simulink model "ProyectoFinal"  (R2024b)
settings: Solver=ode15s  StartTime=0.0  StopTime=10  RelTol=1e-3
undefined symbols (not defined in the file): sigbuilder_block
libraries: slpidlib x1
settings Model: LastModifiedBy=DELL
settings DataIOCC: ReturnWorkspaceOutputs=off  TimeSaveName=t

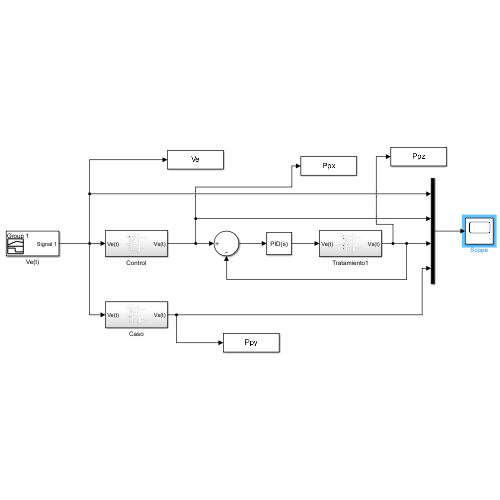
[thumbnail: Simulink's stored preview of the top-level diagram]
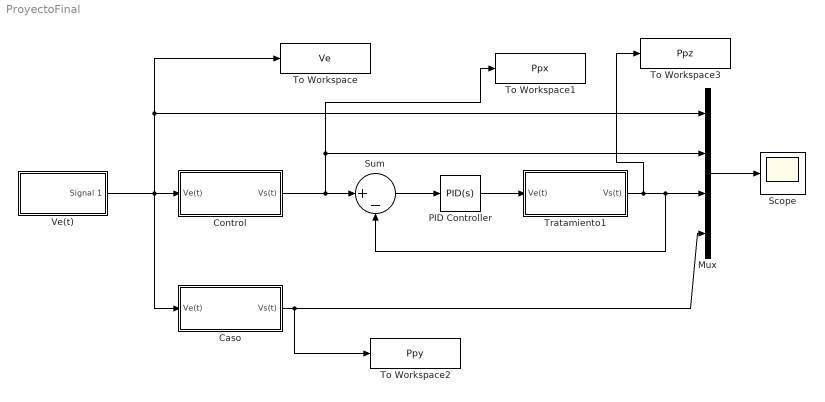
== system ProyectoFinal ==
  Caso : Subsystem
  Control : Subsystem
  Mux : Mux
  PID Controller : slpidlib/PID Controller  Controller=PID  Form=Parallel  TimeDomain=Continuous-time  UseExternalTs=off  SampleTime=-1  IntegratorMethod=Forward Euler  FilterMethod=Forward Euler  ControllerParametersSource=internal  P=8218.94505806436  I=15443765.2569091  UseKiTs=off  D=0.14672186378579  UseExternalDerivativeSource=off  N=0007103298  UseFilter=on  TunerSelectOption=Transfer Function Based (PID Tuner App)  InitialConditionSource=internal  InitialConditionForIntegrator=0  InitialConditionForFilter=0  DifferentiatorICPrevScaledInput=0  ExternalReset=none  TrackingMode=off  Kt=1  LimitOutput=off  SatLimitsSource=internal  UpperSaturationLimit=inf  LowerSaturationLimit=-inf  LinearizeAsGain=on  AntiWindupMode=none  Kb=1  LimitIntegrator=off  UpperIntegratorSaturationLimit=inf  LowerIntegratorSaturationLimit=-inf  POutMin=[]  POutMax=[]  IOutMin=[]  IOutMax=[]  DOutMin=[]  DOutMax=[]  NOutMin=[]  NOutMax=[]  SumOutMin=[]  SumOutMax=[]  SaturationOutMin=[]  SaturationOutMax=[]  PParamMin=[]  PParamMax=[]  IParamMin=[]  IParamMax=[]  DParamMin=[]  DParamMax=[]  NParamMin=[]  NParamMax=[]  KbParamMin=[]  KbParamMax=[]  KtParamMin=[]  KtParamMax=[]  KbOutMin=[]  KbOutMax=[]  KtOutMin=[]  KtOutMax=[]  IntegratorOutMin=[]  IntegratorOutMax=[]  FilterOutMin=[]  FilterOutMax=[]  SumI1OutMin=[]  SumI1OutMax=[]  SumI2OutMin=[]  SumI2OutMax=[]  SumI3OutMin=[]  SumI3OutMax=[]  SumI4OutMin=[]  SumI4OutMax=[]  SumDOutMin=[]  SumDOutMax=[]  DifferentiatorOutMin=[]  DifferentiatorOutMax=[]  FilterDiffOutCoefMin=[]  FilterDiffOutCoefMax=[]  ReciprocalOutMin=[]  ReciprocalOutMax=[]  SumDenOutMin=[]  SumDenOutMax=[]  SumNumOutMin=[]  SumNumOutMax=[]  DivideOutMin=[]  DivideOutMax=[]  UdiffTsProdOutMin=[]  UdiffTsProdOutMax=[]  NTsProdOutMin=[]  NTsProdOutMax=[]  UintegralTsProdOutMin=[]  UintegralTsProdOutMax=[]  UngainTsProdOutMin=[]  UngainTsProdOutMax=[]  ClampingZeroOutDataTypeStr=Inherit: Inherit via back propagation  ClampingZeroOutMin=[]  ClampingZeroOutMax=[]  FilterDenConstantOutDataTypeStr=Inherit: Inherit via back propagation  FilterDenConstantOutMin=[]  FilterDenConstantOutMax=[]  PCopyOutDataTypeStr=Inherit: Inherit via back propagation  PCopyOutMin=[]  PCopyOutMax=[]  NCopyOutDataTypeStr=Inherit: Inherit via back propagation  NCopyOutMin=[]  NCopyOutMax=[]  IntegratorContinuousStateAttributes=''  IntegratorStateMustResolveToSignalObject=off  IntegratorRTWStateStorageClass=Auto  FilterContinuousStateAttributes=''  FilterStateMustResolveToSignalObject=off  FilterRTWStateStorageClass=Auto  ParallelPVariant=InternalParameters  IdealPVariant=Disabled  IVariant=InternalParameters  DVariant=InternalParameters  IntegratorVariant=Continuous  SatVariant=Disabled  AWVariant=Passthrough  PCopyVariant=Disabled  TRVariant=Disabled  FdbkBlocksVariant=Forward  IdealPFdbkVariant=Disabled  SatFdbkVariant=Disabled  DerivativeFilterVariant=ContFilter  NVariant=InternalParameters  NCopyVariant=Disabled  FilterICVariant=InternalICsFilter  IntegratorICVariant=InternalICs  ExternalResetVariant=Disabled  TRSumVariant=Passthrough  SumFdbkVariant=Disabled  SumVariant=Sum_PID  TsampFilterVariant=InternalTs  TsampNgainVariant=Passthrough  TsampIntegralVariant=Disabled_SignalSpec  ExternalSaturationOutDataTypeStr=Inherit: Same as second input  DerivativeSourceVariant=ErrorSignal  PreIntVariant=InternalPreInt
  Scope : Scope
  Sum : Sum  Inputs=|+-
  To Workspace : ToWorkspace  VariableName=Ve  SaveFormat=Timeseries  SampleTime=-1
  To Workspace1 : ToWorkspace  VariableName=Ppx  SaveFormat=Timeseries  SampleTime=-1
  To Workspace2 : ToWorkspace  VariableName=Ppy  SaveFormat=Timeseries  SampleTime=-1
  To Workspace3 : ToWorkspace  VariableName=Ppz  SaveFormat=Timeseries  SampleTime=-1
  Tratamiento1 : Subsystem
  Ve(t) : Subsystem  Tag=STV Subsys  LoadFcn=sigbuilder_block('load');  StartFcn=sigbuilder_block('start');  StopFcn=sigbuilder_block('stop');  ClipboardFcn=sigbuilder_block('clipboard');  mask(Sigbuilder block){tuvar=[0:10]}
      mask help: Simulink:masks:SigbuilderBlock_MD
      mask init:
      | if ~strcmp(get_param(bdroot(gcbh),'SimulationStatus'),'stopped') tuvar = sigbuilder_block('maskInit'); end
      settings: CopyFcn=sigbuilder_block('copy');  DeleteFcn=sigbuilder_block('delete');  ModelCloseFcn=sigbuilder_block('modelClose');  PreSaveFcn=sigbuilder_block('preSave');  PauseFcn=sigbuilder_block('pause');  ContinueFcn=sigbuilder_block('continue');  NameChangeFcn=sigbuilder_block('namechange');  OpenFcn=sigbuilder_block('open',[437.6 199.2 550.4 400 ]);  CloseFcn=sigbuilder_block('close');
      mask Display: plot(0, 0, 100, 100,[2, 2, 32, 32, 2], [68, 8, 8, 68, 68],[32, 2], [38, 38], [32, 19, 2],[53, 60, 44], [32, 17, 17, 2],[16, 16, 31, 31]);txt = getActiveGroup(gcbh);text(2, 100, txt,'verticalAlignment', 'top');
  wires:
  Control/1(Vs(t)) -> Mux/2, To Workspace1/1, Sum/1
  Mux/1 -> Scope/1
  Caso/1(Vs(t)) -> To Workspace2/1, Mux/4
  Tratamiento1/1(Vs(t)) -> To Workspace3/1, Mux/3, Sum/2
  Sum/1 -> PID Controller/1
  PID Controller/1 -> Tratamiento1/1(Ve(t))
  Ve(t)/1(Signal 1) -> Caso/1(Ve(t)), Control/1(Ve(t)), To Workspace/1, Mux/1

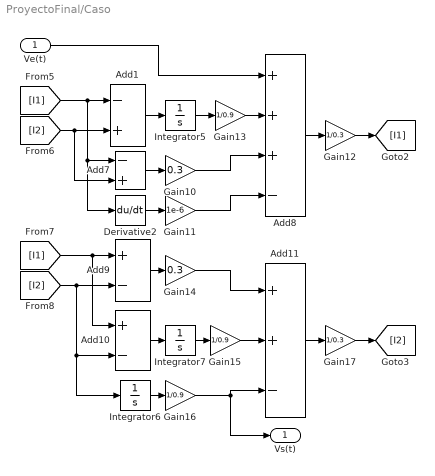
== system ProyectoFinal/Caso ==
  Ve(t) : Inport
  Add1 : Sum  Inputs=-+
  Add10 : Sum  Inputs=+-
  Add11 : Sum  Inputs=++-
  Add7 : Sum  Inputs=-+
  Add8 : Sum  Inputs=+++-
  Add9 : Sum  Inputs=+-
  Derivative2 : Derivative
  Gain10 : Gain  Gain=0.3
  Gain11 : Gain  Gain=1e-6
  Gain12 : Gain  Gain=1/0.3
  Gain13 : Gain  Gain=1/0.9
  Gain14 : Gain  Gain=0.3
  Gain15 : Gain  Gain=1/0.9
  Gain16 : Gain  Gain=1/0.9
  Gain17 : Gain  Gain=1/0.3
  Integrator5 : Integrator
  Integrator6 : Integrator
  Integrator7 : Integrator
  Vs(t) : Outport
  wires:
  Add8/1 -> Gain12/1
  Integrator6/1 -> Gain16/1
  Gain17/1 -> [I2]
  Integrator7/1 -> Gain15/1
  Add11/1 -> Gain17/1
  Gain10/1 -> Add8/3
  Add10/1 -> Integrator7/1
  Gain13/1 -> Add8/2
  Derivative2/1 -> Gain11/1
  Integrator5/1 -> Gain13/1
  Gain11/1 -> Add8/4
  Gain16/1 -> Vs(t)/1, Add11/3
  Add1/1 -> Integrator5/1
  [I2] -> Integrator6/1, Add10/2, Add9/2
  [I1] -> Add10/1, Add9/1
  [I1] -> Add1/1, Derivative2/1, Add7/1
  Gain14/1 -> Add11/1
  Gain15/1 -> Add11/2
  Add7/1 -> Gain10/1
  Gain12/1 -> [I1]
  Add9/1 -> Gain14/1
  [I2] -> Add1/2, Add7/2
  Ve(t)/1 -> Add8/1

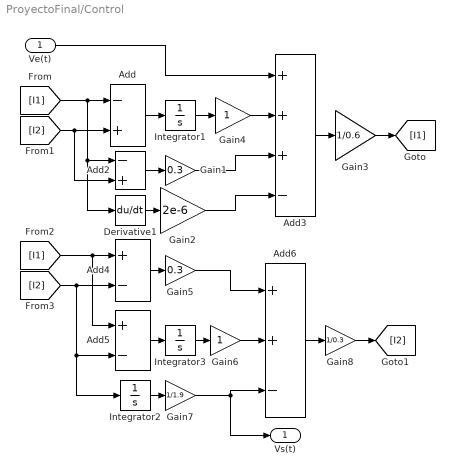
== system ProyectoFinal/Control ==
  Ve(t) : Inport
  Add : Sum  Inputs=-+
  Add2 : Sum  Inputs=-+
  Add3 : Sum  Inputs=+++-
  Add4 : Sum  Inputs=+-
  Add5 : Sum  Inputs=+-
  Add6 : Sum  Inputs=++-
  Derivative1 : Derivative
  Gain1 : Gain  Gain=0.3
  Gain2 : Gain  Gain=2e-6
  Gain3 : Gain  Gain=1/0.6
  Gain4 : Gain
  Gain5 : Gain  Gain=0.3
  Gain6 : Gain
  Gain7 : Gain  Gain=1/1.9
  Gain8 : Gain  Gain=1/0.3
  Integrator1 : Integrator
  Integrator2 : Integrator
  Integrator3 : Integrator
  Vs(t) : Outport
  wires:
  [I1] -> Add/1, Derivative1/1, Add2/1
  [I2] -> Add/2, Add2/2
  Add2/1 -> Gain1/1
  Add/1 -> Integrator1/1
  Derivative1/1 -> Gain2/1
  Ve(t)/1 -> Add3/1
  Gain1/1 -> Add3/3
  Gain2/1 -> Add3/4
  Add3/1 -> Gain3/1
  Gain3/1 -> [I1]
  Integrator1/1 -> Gain4/1
  Gain4/1 -> Add3/2
  [I1] -> Add5/1, Add4/1
  [I2] -> Integrator2/1, Add5/2, Add4/2
  Add4/1 -> Gain5/1
  Integrator3/1 -> Gain6/1
  Integrator2/1 -> Gain7/1
  Gain5/1 -> Add6/1
  Gain6/1 -> Add6/2
  Gain7/1 -> Vs(t)/1, Add6/3
  Add5/1 -> Integrator3/1
  Add6/1 -> Gain8/1
  Gain8/1 -> [I2]

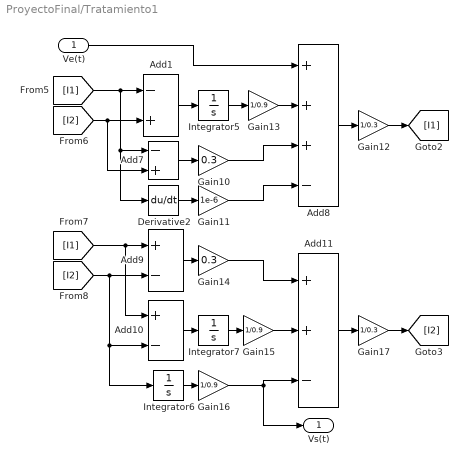
== system ProyectoFinal/Tratamiento1 ==
  Ve(t) : Inport
  Add1 : Sum  Inputs=-+
  Add10 : Sum  Inputs=+-
  Add11 : Sum  Inputs=++-
  Add7 : Sum  Inputs=-+
  Add8 : Sum  Inputs=+++-
  Add9 : Sum  Inputs=+-
  Derivative2 : Derivative
  Gain10 : Gain  Gain=0.3
  Gain11 : Gain  Gain=1e-6
  Gain12 : Gain  Gain=1/0.3
  Gain13 : Gain  Gain=1/0.9
  Gain14 : Gain  Gain=0.3
  Gain15 : Gain  Gain=1/0.9
  Gain16 : Gain  Gain=1/0.9
  Gain17 : Gain  Gain=1/0.3
  Integrator5 : Integrator
  Integrator6 : Integrator
  Integrator7 : Integrator
  Vs(t) : Outport
  wires:
  Ve(t)/1 -> Add8/1
  Gain12/1 -> [I1]
  [I2] -> Add1/2, Add7/2
  Add7/1 -> Gain10/1
  Gain14/1 -> Add11/1
  Gain15/1 -> Add11/2
  [I1] -> Add1/1, Derivative2/1, Add7/1
  [I2] -> Integrator6/1, Add10/2, Add9/2
  [I1] -> Add10/1, Add9/1
  Gain16/1 -> Vs(t)/1, Add11/3
  Integrator5/1 -> Gain13/1
  Add1/1 -> Integrator5/1
  Gain13/1 -> Add8/2
  Gain11/1 -> Add8/4
  Derivative2/1 -> Gain11/1
  Add9/1 -> Gain14/1
  Gain17/1 -> [I2]
  Add11/1 -> Gain17/1
  Add10/1 -> Integrator7/1
  Gain10/1 -> Add8/3
  Integrator7/1 -> Gain15/1
  Integrator6/1 -> Gain16/1
  Add8/1 -> Gain12/1

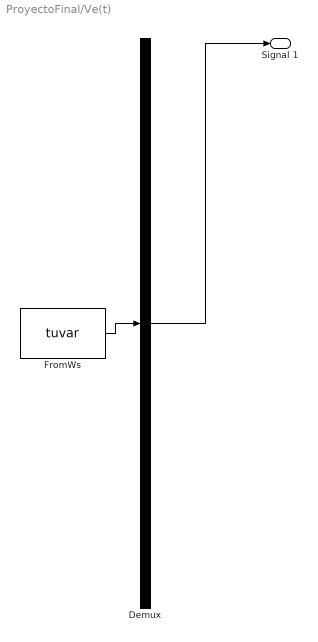
== system ProyectoFinal/Ve(t) ==
  Demux : Demux  Tag=STV Demux  Outputs=1
      settings: DisplayOption=none
  FromWs : FromWorkspace  Tag=STV FromWs  VariableName=tuvar
      SigBuilderData=|
      | common.afterFinalStr = 'Extrapolate'
      | common.sampleTime = 0
      | dataSet.timeRange = [0 10]
      | dataSet.name = 'Group 1'
      | sbobj.Groups.Name = 'Group 1'
      | sbobj.Groups.Signals.Name = 'Signal 1'
      | sbobj.Groups.Signals.XData = [0 9 10]
      | sbobj.Groups.Signals.YData = [0 1 0]
  Signal 1 : Outport  Tag=STV Outport
  wires:
  Demux/1 -> Signal 1/1
  FromWs/1 -> Demux/1
